simulink model "Hit_Crossing"  (Simulink 8.0)
settings: Solver=ode45  StartTime=0.0  StopTime=6  RelTol=1e-3
settings Model: Creator=Faradars  LastModifiedBy=Faradars

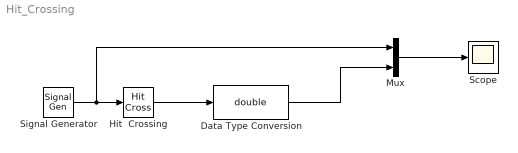
== system Hit_Crossing ==
  Data Type Conversion : DataTypeConversion  OutDataTypeStr=double
  Hit  Crossing : HitCross  HitCrossingOffset=-1
  Mux : Mux  Inputs=2
  Scope : Scope
  Signal Generator : SignalGenerator  Frequency=0.25
  wires:
  Mux/1 -> Scope/1
  Signal Generator/1 -> Mux/1, Hit  Crossing/1
  Hit  Crossing/1 -> Data Type Conversion/1
  Data Type Conversion/1 -> Mux/2
